simulink model "sampleModel106"  (R2021b)
settings: Solver=VariableStepAuto  StartTime=0.0  StopTime=10.0  RelTol=1e-3
libraries: simulink x2
settings Model: Creator=user  LastModifiedBy=user

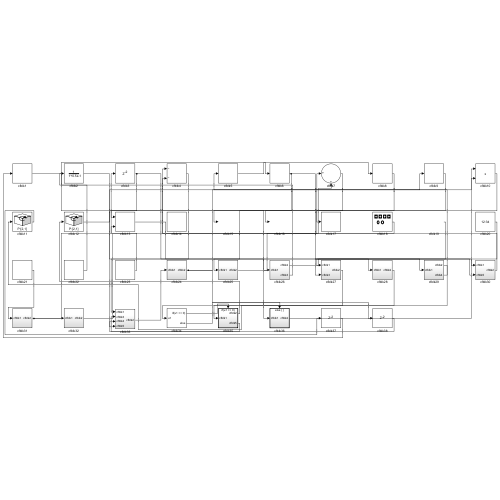
[thumbnail: Simulink's stored preview of the top-level diagram]
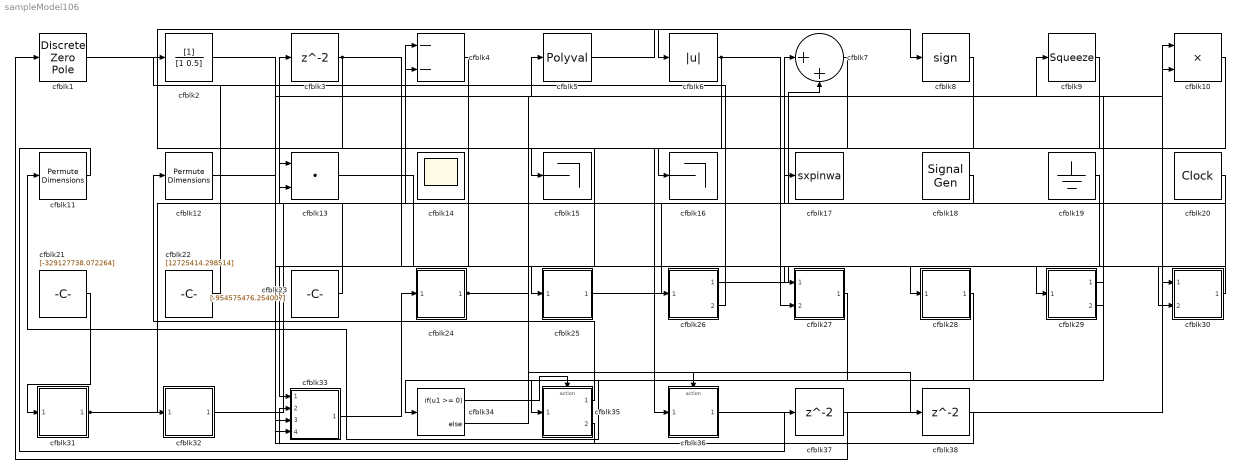
== system sampleModel106 ==
  cfblk1 : DiscreteZeroPole  Poles=[0 0.5]  Gain=1
  cfblk10 : Product  Inputs=**
  cfblk11 : PermuteDimensions
  cfblk12 : PermuteDimensions
  cfblk13 : DotProduct  InputSameDT=on  OutDataTypeStr=Inherit: Inherit via internal rule
  cfblk14 : Scope
      settings: Floating=on
  cfblk15 : Terminator
  cfblk16 : Terminator
  cfblk17 : ToWorkspace  VariableName=sxpinwa  SaveFormat=Timeseries  SampleTime=-1
  cfblk18 : SignalGenerator  WaveForm=sawtooth  Amplitude=[174804602.650476]  Units=rad/sec
  cfblk19 : Ground
  cfblk2 : DiscreteFilter  SampleTime=1
  cfblk20 : DigitalClock
  cfblk21 : Constant  Value=[-329127738.072264]  SampleTime=1
  cfblk22 : Constant  Value=[12725414.298514]  SampleTime=1
  cfblk23 : Constant  Value=[-954575476.254007]  SampleTime=1
  cfblk24 : Subsystem
  cfblk25 : Subsystem
  cfblk26 : Subsystem
  cfblk27 : Subsystem
  cfblk28 : Subsystem
  cfblk29 : Subsystem
  cfblk3 : Delay  SampleTime=1
  cfblk30 : Subsystem
  cfblk31 : Subsystem
  cfblk32 : Subsystem
  cfblk33 : Subsystem
  cfblk34 : If  IfExpression=u1 >= 0  SampleTime=1
  cfblk35 : Subsystem  TreatAsAtomicUnit=on
  cfblk36 : Subsystem  TreatAsAtomicUnit=on
  cfblk37 : Delay  SampleTime=1
  cfblk38 : Delay  SampleTime=1
  cfblk4 : Sum  Inputs=--
  cfblk5 : Polyval  Coefs=[ +2.081618890e-019, -1.441693666e-014, +4.719686976e-010, -8.536869453e-006, +1.621573104e-001, -8.087801117e+001 ]
  cfblk6 : Abs
  cfblk7 : Sum  Inputs=|++
  cfblk8 : Signum
  cfblk9 : Squeeze
  wires:
  cfblk36/1(cfblk2) -> cfblk10/1
  cfblk9/1 -> cfblk15/1
  cfblk35/1(cfblk2) -> cfblk12/1
  cfblk18/1 -> cfblk4/1
  cfblk26/1(cfblk2) -> cfblk29/1(cfblk1)
  cfblk20/1 -> cfblk27/1(cfblk1)
  cfblk23/1 -> cfblk3/1
  cfblk29/1(cfblk2) -> cfblk11/1
  cfblk2/1 -> cfblk30/1(cfblk1)
  cfblk10/1 -> cfblk25/1(cfblk1)
  cfblk6/1 -> cfblk13/1, cfblk30/2(cfblk5)
  cfblk22/1 -> cfblk6/1
  cfblk5/1 -> cfblk8/1
  cfblk27/1(cfblk2) -> cfblk35/1(cfblk1)
  cfblk21/1 -> cfblk31/1(cfblk1)
  cfblk28/1(cfblk2) -> cfblk34/1
  cfblk7/1 -> cfblk16/1
  cfblk19/1 -> cfblk27/2(cfblk3)
  cfblk30/1(cfblk2) -> cfblk4/2
  cfblk33/1(cfblk2) -> cfblk24/1(cfblk1)
  cfblk25/1(cfblk2) -> cfblk7/1
  cfblk1/1 -> cfblk26/1(cfblk1)
  cfblk3/1 -> cfblk28/1(cfblk1), cfblk33/4(cfblk5)
  cfblk31/1(cfblk2) -> cfblk13/2, cfblk32/1(cfblk1)
  cfblk32/1(cfblk2) -> cfblk7/2
  cfblk4/1 -> cfblk33/1(cfblk1)
  cfblk24/1(cfblk2) -> cfblk9/1, cfblk38/1
  cfblk35/2(cfblk5) -> cfblk33/2(cfblk3)
  cfblk12/1 -> cfblk10/2
  cfblk13/1 -> cfblk36/1(cfblk1)
  cfblk8/1 -> cfblk17/1
  cfblk26/2(cfblk3) -> cfblk2/1
  cfblk29/2(cfblk4) -> cfblk5/1
  cfblk34/1 -> cfblk35/Action
  cfblk34/2 -> cfblk36/Action
  cfblk11/1 -> cfblk37/1
  cfblk37/1 -> cfblk1/1
  cfblk38/1 -> cfblk33/3(cfblk4)

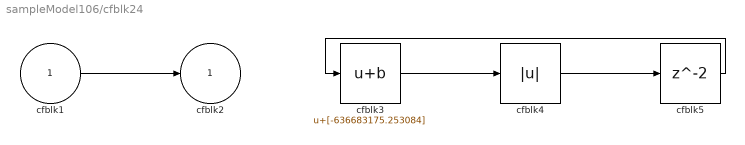
== system sampleModel106/cfblk24 ==
  cfblk1 : Inport
  cfblk3 : Bias  Bias=[-636683175.253084]
  cfblk4 : Abs
  cfblk5 : Delay  SampleTime=1
  cfblk2 : Outport
  wires:
  cfblk1/1 -> cfblk2/1
  cfblk3/1 -> cfblk4/1
  cfblk4/1 -> cfblk5/1
  cfblk5/1 -> cfblk3/1

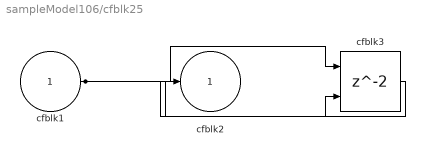
== system sampleModel106/cfblk25 ==
  cfblk1 : Inport
  cfblk3 : Delay  ShowEnablePort=on  SampleTime=1
      settings: InputPortMap=u0,e6
  cfblk2 : Outport
  wires:
  cfblk1/1 -> cfblk3/1, cfblk3/2
  cfblk3/1 -> cfblk2/1

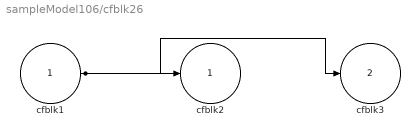
== system sampleModel106/cfblk26 ==
  cfblk1 : Inport
  cfblk2 : Outport
  cfblk3 : Outport  Port=2
  wires:
  cfblk1/1 -> cfblk2/1, cfblk3/1

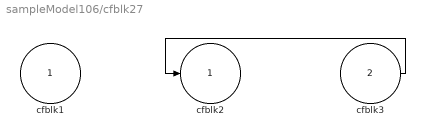
== system sampleModel106/cfblk27 ==
  cfblk1 : Inport
  cfblk3 : Inport  Port=2
  cfblk2 : Outport
  wires:
  cfblk3/1 -> cfblk2/1

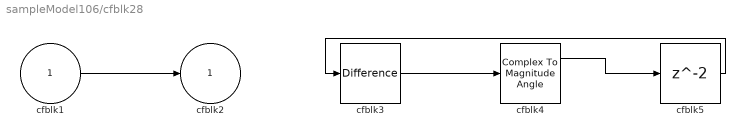
== system sampleModel106/cfblk28 ==
  cfblk1 : Inport
  cfblk3 : simulink/Discrete/Difference  ICPrevInput=0.0  OutMin=[]  OutMax=[]  OutDataTypeStr=Inherit: Inherit via back propagation  OutDataType=fixdt(1, 16)  OutScaling=2^-10  DoSatur=off
  cfblk4 : ComplexToMagnitudeAngle
  cfblk5 : Delay  SampleTime=1
  cfblk2 : Outport
  wires:
  cfblk1/1 -> cfblk2/1
  cfblk3/1 -> cfblk4/1
  cfblk4/1 -> cfblk5/1
  cfblk5/1 -> cfblk3/1

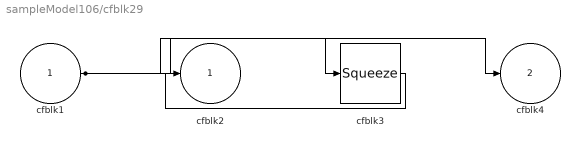
== system sampleModel106/cfblk29 ==
  cfblk1 : Inport
  cfblk3 : Squeeze
  cfblk2 : Outport
  cfblk4 : Outport  Port=2
  wires:
  cfblk1/1 -> cfblk4/1, cfblk3/1
  cfblk3/1 -> cfblk2/1

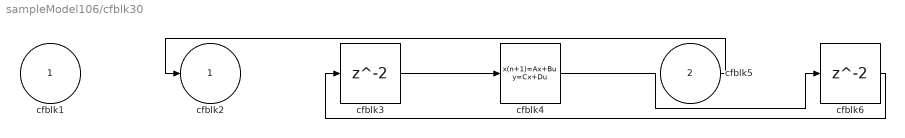
== system sampleModel106/cfblk30 ==
  cfblk1 : Inport
  cfblk5 : Inport  Port=2
  cfblk3 : Delay  SampleTime=1
  cfblk4 : DiscreteStateSpace
  cfblk6 : Delay  SampleTime=1
  cfblk2 : Outport
  wires:
  cfblk5/1 -> cfblk2/1
  cfblk3/1 -> cfblk4/1
  cfblk4/1 -> cfblk6/1
  cfblk6/1 -> cfblk3/1

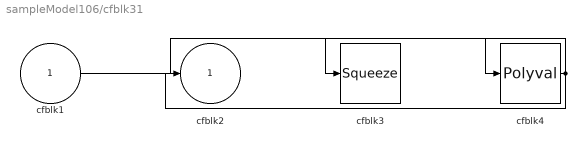
== system sampleModel106/cfblk31 ==
  cfblk1 : Inport
  cfblk3 : Squeeze
  cfblk4 : Polyval  Coefs=[ +2.081618890e-019, -1.441693666e-014, +4.719686976e-010, -8.536869453e-006, +1.621573104e-001, -8.087801117e+001 ]
  cfblk2 : Outport
  wires:
  cfblk1/1 -> cfblk4/1
  cfblk4/1 -> cfblk2/1, cfblk3/1

== system sampleModel106/cfblk32 ==
  cfblk1 : Inport
  cfblk3 : simulink/Math Operations/MinMax Running Resettable  Function=min  vinit=0.0
  cfblk2 : Outport
  wires:
  cfblk1/1 -> cfblk3/1, cfblk3/2
  cfblk3/1 -> cfblk2/1

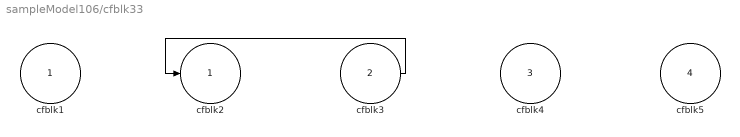
== system sampleModel106/cfblk33 ==
  cfblk1 : Inport
  cfblk3 : Inport  Port=2
  cfblk4 : Inport  Port=3
  cfblk5 : Inport  Port=4
  cfblk2 : Outport
  wires:
  cfblk3/1 -> cfblk2/1

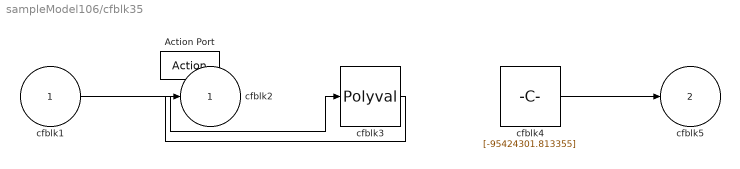
== system sampleModel106/cfblk35 ==
  cfblk1 : Inport
  Action Port : ActionPort  ActionPortLabel=if(u1 >= 0)
  cfblk3 : Polyval  Coefs=[ +2.081618890e-019, -1.441693666e-014, +4.719686976e-010, -8.536869453e-006, +1.621573104e-001, -8.087801117e+001 ]
  cfblk4 : Constant  Value=[-95424301.813355]  SampleTime=1
  cfblk2 : Outport
  cfblk5 : Outport  Port=2
  wires:
  cfblk4/1 -> cfblk5/1
  cfblk1/1 -> cfblk3/1
  cfblk3/1 -> cfblk2/1

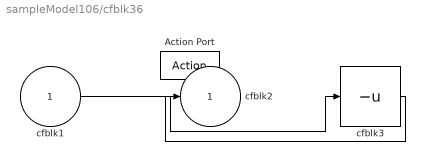
== system sampleModel106/cfblk36 ==
  cfblk1 : Inport
  Action Port : ActionPort  ActionPortLabel=else
  cfblk3 : UnaryMinus
  cfblk2 : Outport
  wires:
  cfblk1/1 -> cfblk3/1
  cfblk3/1 -> cfblk2/1
